simulink model "Switching_controller_with_noise"  (R2019b)
settings: Solver=VariableStepAuto  StartTime=0.0  StopTime=10.0  RelTol=1e-3
libraries: simulink x1
settings Model: Creator=chint  LastModifiedBy=chint

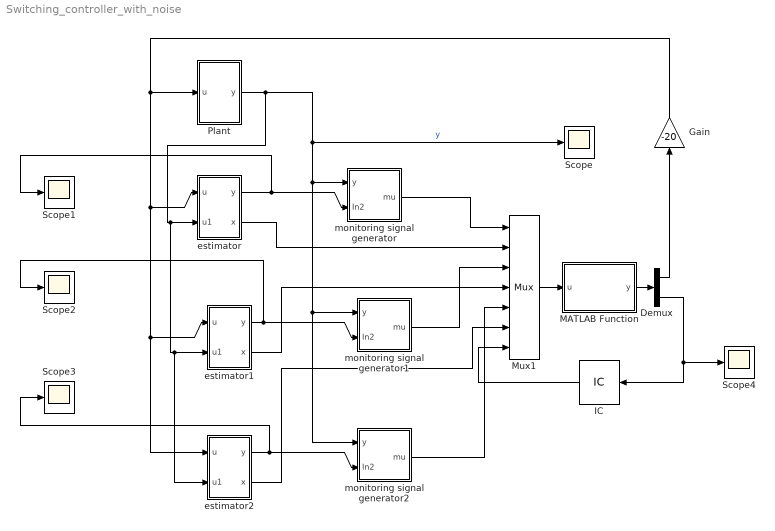
== system Switching_controller_with_noise ==
  Demux : Demux  Outputs=2
  Gain : Gain  Gain=-20
  IC : InitialCondition  Value=3
  MATLAB Function : MATLAB Function  TreatAsAtomicUnit=on
  Mux1 : Mux  Inputs=7
  Plant : Subsystem
  Scope{,1..4} (5 alike) : Scope
  estimator : Subsystem
  estimator1 : Subsystem
  estimator2 : Subsystem
  monitoring signal generator : Subsystem
  monitoring signal generator1 : Subsystem
  monitoring signal generator2 : Subsystem
  wires:
  estimator/1(y) -> Scope1/1, monitoring signal generator/2(In2)
  monitoring signal generator/1(mu) -> Mux1/1
  estimator1/1(y) -> Scope2/1, monitoring signal generator1/2(In2)
  monitoring signal generator1/1(mu) -> Mux1/3
  Gain/1 -> estimator2/1(u), estimator1/1(u), estimator/1(u), Plant/1(u)
  Plant/1(y) -> estimator2/2(u1), estimator1/2(u1), estimator/2(u1), Scope/1, monitoring signal generator2/1(y), monitoring signal generator1/1(y), monitoring signal generator/1(y)  "y"
  monitoring signal generator2/1(mu) -> Mux1/5
  estimator2/1(y) -> Scope3/1, monitoring signal generator2/2(In2)
  estimator/2(x) -> Mux1/2
  estimator1/2(x) -> Mux1/4
  estimator2/2(x) -> Mux1/6
  Mux1/1 -> MATLAB Function/1(u)
  MATLAB Function/1(y) -> Demux/1
  Demux/1 -> Gain/1
  Demux/2 -> Scope4/1, IC/1
  IC/1 -> Mux1/7

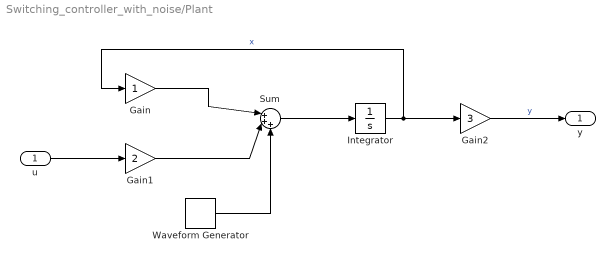
== system Switching_controller_with_noise/Plant ==
  u : Inport
  Gain : Gain
  Gain1 : Gain  Gain=2
  Gain2 : Gain  Gain=3
  Integrator : Integrator  InitialCondition=10
  Sum : Sum  Inputs=|+++
  Waveform Generator : simulink/Sources/Waveform Generator  OutMin=[]  OutMax=[]  OutDataTypeStr=double  SelectedSignal=1  Signals=sin(2,3,1)  BlockNames=MultiportSwitch_10d59e586fcb425  SampleTime=0.1
      settings: SourceProductName=Simulink
  y : Outport
  wires:
  Integrator/1 -> Gain2/1, Gain/1  "x"
  u/1 -> Gain1/1
  Gain1/1 -> Sum/2
  Gain2/1 -> y/1  "y"
  Sum/1 -> Integrator/1
  Gain/1 -> Sum/1
  Waveform Generator/1 -> Sum/3

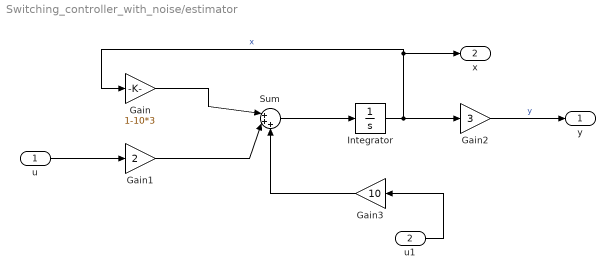
== system Switching_controller_with_noise/estimator ==
  u : Inport
  u1 : Inport  Port=2
  Gain : Gain  Gain=1-10*3
  Gain1 : Gain  Gain=2
  Gain2 : Gain  Gain=3
  Gain3 : Gain  Gain=10
  Integrator : Integrator
  Sum : Sum  Inputs=|+++
  y : Outport
  x : Outport  Port=2
  wires:
  Integrator/1 -> Gain2/1, x/1, Gain/1  "x"
  u/1 -> Gain1/1
  Gain1/1 -> Sum/2
  Gain2/1 -> y/1  "y"
  Sum/1 -> Integrator/1
  Gain/1 -> Sum/1
  Gain3/1 -> Sum/3
  u1/1 -> Gain3/1

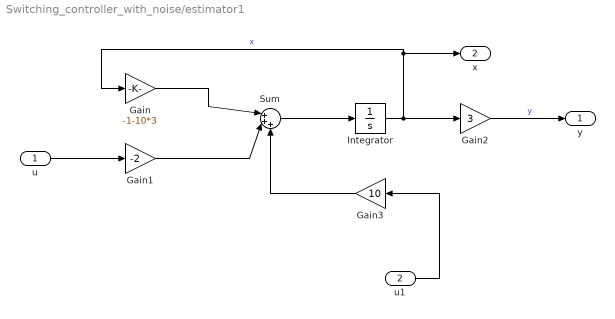
== system Switching_controller_with_noise/estimator1 ==
  u : Inport
  u1 : Inport  Port=2
  Gain : Gain  Gain=-1-10*3
  Gain1 : Gain  Gain=-2
  Gain2 : Gain  Gain=3
  Gain3 : Gain  Gain=10
  Integrator : Integrator
  Sum : Sum  Inputs=|+++
  y : Outport
  x : Outport  Port=2
  wires:
  Integrator/1 -> Gain2/1, x/1, Gain/1  "x"
  u/1 -> Gain1/1
  Gain1/1 -> Sum/2
  Gain2/1 -> y/1  "y"
  Sum/1 -> Integrator/1
  Gain/1 -> Sum/1
  Gain3/1 -> Sum/3
  u1/1 -> Gain3/1

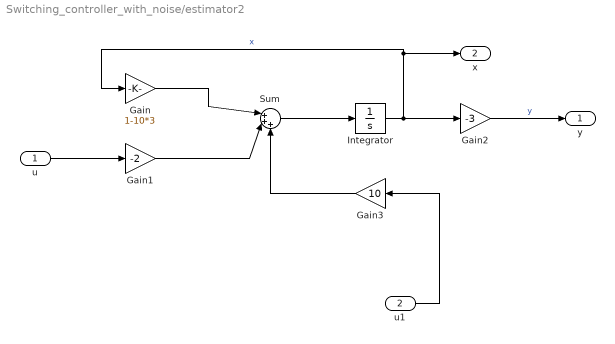
== system Switching_controller_with_noise/estimator2 ==
  u : Inport
  u1 : Inport  Port=2
  Gain : Gain  Gain=1-10*3
  Gain1 : Gain  Gain=-2
  Gain2 : Gain  Gain=-3
  Gain3 : Gain  Gain=10
  Integrator : Integrator
  Sum : Sum  Inputs=|+++
  y : Outport
  x : Outport  Port=2
  wires:
  Integrator/1 -> Gain2/1, x/1, Gain/1  "x"
  u/1 -> Gain1/1
  Gain1/1 -> Sum/2
  Gain2/1 -> y/1  "y"
  Sum/1 -> Integrator/1
  Gain/1 -> Sum/1
  Gain3/1 -> Sum/3
  u1/1 -> Gain3/1

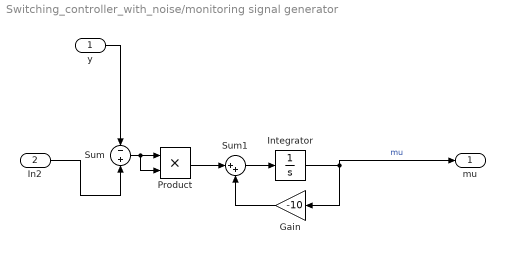
== system Switching_controller_with_noise/monitoring signal generator ==
  y : Inport
  In2 : Inport  Port=2
  Gain : Gain  Gain=-10
  Integrator : Integrator
  Product : Product
  Sum : Sum  Inputs=-+
  Sum1 : Sum  Inputs=|++
  mu : Outport
  wires:
  Integrator/1 -> mu/1, Gain/1  "mu"
  Sum1/1 -> Integrator/1
  y/1 -> Sum/1
  Sum/1 -> Product/2, Product/1
  In2/1 -> Sum/2
  Product/1 -> Sum1/1
  Gain/1 -> Sum1/2

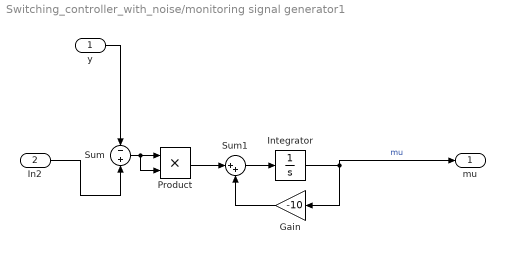
== system Switching_controller_with_noise/monitoring signal generator1 ==
  y : Inport
  In2 : Inport  Port=2
  Gain : Gain  Gain=-10
  Integrator : Integrator
  Product : Product
  Sum : Sum  Inputs=-+
  Sum1 : Sum  Inputs=|++
  mu : Outport
  wires:
  Integrator/1 -> mu/1, Gain/1  "mu"
  Sum1/1 -> Integrator/1
  y/1 -> Sum/1
  Sum/1 -> Product/2, Product/1
  In2/1 -> Sum/2
  Product/1 -> Sum1/1
  Gain/1 -> Sum1/2

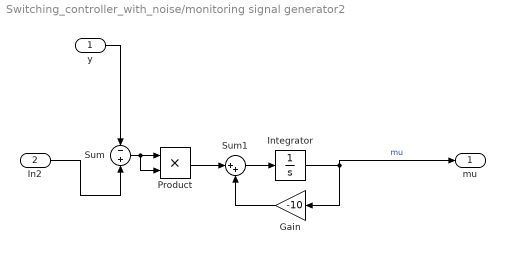
== system Switching_controller_with_noise/monitoring signal generator2 ==
  y : Inport
  In2 : Inport  Port=2
  Gain : Gain  Gain=-10
  Integrator : Integrator
  Product : Product
  Sum : Sum  Inputs=-+
  Sum1 : Sum  Inputs=|++
  mu : Outport
  wires:
  Integrator/1 -> mu/1, Gain/1  "mu"
  Sum1/1 -> Integrator/1
  y/1 -> Sum/1
  Sum/1 -> Product/2, Product/1
  In2/1 -> Sum/2
  Product/1 -> Sum1/1
  Gain/1 -> Sum1/2

== matlab function Switching_controller_with_noise/MATLAB Function ==
  data: u input; y output
function y = fcn(u)
   [l,m]=min([u(1);u(3);u(5)]);
   h=10;
   if l+h<u(int64(2*u(7)-1))
       y=[u(2*m);m];
   else
       y=[u(2*u(7));u(7)];
   end
end
